simulink model "prob3_week2"  (R2020b)
settings: Solver=VariableStepAuto  StartTime=0.0  StopTime=10.0  RelTol=1e-3
undefined symbols (not defined in the file): b, m
settings Model: Creator=Pulkit Khandelwal  LastModifiedBy=Pulkit Khandelwal

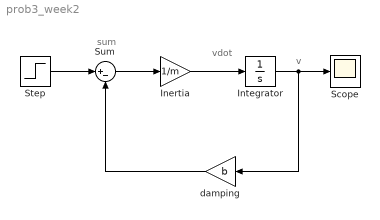
== system prob3_week2 ==
  note: v
  note: sum
  note: vdot
  Inertia : Gain  Gain=1/m
  Integrator : Integrator
  Scope : Scope
  Step : Step  SampleTime=0
  Sum : Sum  Inputs=|+-
  damping : Gain  Gain=b
  wires:
  damping/1 -> Sum/2
  Step/1 -> Sum/1
  Sum/1 -> Inertia/1
  Integrator/1 -> Scope/1, damping/1
  Inertia/1 -> Integrator/1
